simulink model "Reformable_AI"  (R2026a)
settings: Solver=ode23t  StopTime=10  FixedStep=0.01
InitFcn:
  | load('PV_Params_Stage1.mat'); load('PV_Params_Stage2.mat');
values from neighbouring files (symbols this model uses):
  Eg = 1.12    [PV_Params_Stage1.mat]    (also in reformable_AI.m)
  Gref = 1000    [PV_Params_Stage1.mat]    (also in reformable_AI.m)
  I0_ref = 3.04931718656e-08    [PV_Params_Stage1.mat]    (also in reformable_AI.m = exp(x_sol(3)))
  Iph_ref = 1.82004673012    [PV_Params_Stage1.mat]    (also in reformable_AI.m = x_sol(2))
  k_Iph = 0.2    [PV_Params_Stage2.mat]    (also in reformable_AI.m)
  k_Q = 0.2    [reformable_AI.m]
  k_R0 = 0.5    [reformable_AI.m]
  k_R1 = 0.6    [reformable_AI.m]
  k_Rs = 0.5    [PV_Params_Stage2.mat]    (also in reformable_AI.m)
  k_Rsh = 0.6    [PV_Params_Stage2.mat]    (also in reformable_AI.m)
  Ki = 0.0006    [PV_Params_Stage1.mat]    (also in reformable_AI.m)
  n = 1.3    [PV_Params_Stage1.mat]    (also in reformable_AI.m)
  Ns = 36    [PV_Params_Stage1.mat]    (also in reformable_AI.m)
  OCV_tbl = [11.6 11.8 11.9 12.1 12.2 12.3 12.4 12.5 12.6 12.7 12.8]    [Battery_Param_Definition.m]    (also in Battery_Params_Stage3.mat; reformable_AI.m)
  Q = 7    [Battery_Param_Definition.m]    (also in Battery_Params_Stage3.mat; reformable_AI.m)
  R0 = 0.03    [Battery_Param_Definition.m]    (also in Battery_Params_Stage3.mat; reformable_AI.m)
  R1 = 0.015    [Battery_Param_Definition.m]    (also in Battery_Params_Stage3.mat; reformable_AI.m)
  Rs = 0.0128377802072    [PV_Params_Stage1.mat]    (also in reformable_AI.m = x(1))
  Rsh = 500    [PV_Params_Stage1.mat]    (also in reformable_AI.m)
  SOC_bp = [0 10 20 30 40 50 60 70 80 90 100]    [Battery_Param_Definition.m]    (also in Battery_Params_Stage3.mat; reformable_AI.m)
  SOC_init = 100    [Battery_Param_Definition.m]    (also in Battery_Params_Stage3.mat; reformable_AI.m)
  T_life = 25    [PV_Params_Stage2.mat]    (also in reformable_AI.m)
  T_life_batt = 10    [reformable_AI.m]
  Tref = 298.15    [PV_Params_Stage1.mat]    (also in reformable_AI.m)
libraries: fl_lib x6, nesl_utility x5, ee_lib_for_power_systems x1
settings Model: Creator=inspiredkhalid  LastModifiedBy=inspiredkhalid

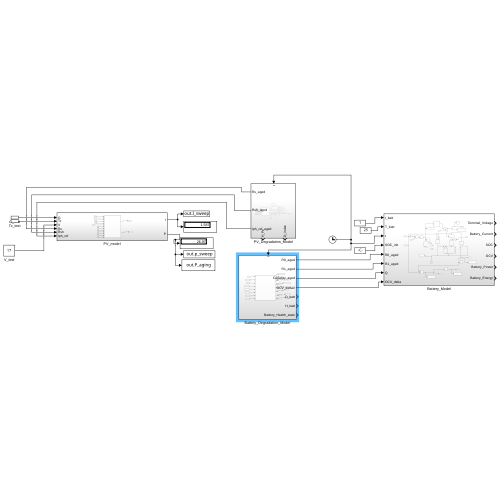
[thumbnail: Simulink's stored preview of the top-level diagram]
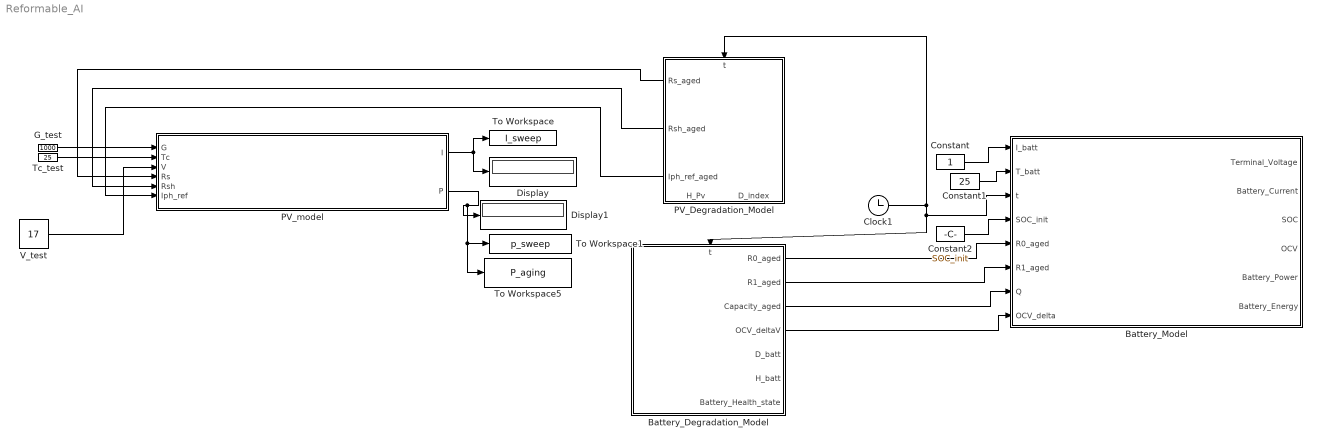
== system Reformable_AI ==
  Battery_Degradation_Model : Subsystem
      settings: PortSchema="{\"entries\":[{\"content\":{\"sides\":[{\"content\":{},\"type\":\"ConnectorPlacement.EquallySpacedRectSide\",\"uuid\":\"1b4fcb6b-66e9-48a9-b94c-f37550c0d7a8\"},{\"content\":{\"connectorIds\":[\"Out1\",\"Out2\",\"Out3\",\"Out4\",\"Out5\",\"Out6\",\"Out7\"],\"side\":\"RIGHT\"},\"type\":\"ConnectorPlacement.EquallySpacedRectSide\",\"uuid\":\"dcdb6d26-adba-4e3a-bfcc-7c50a5c7991f\"},{\"content\":{\"connectorIds\":[\"In1\"],\"side\":\"TOP\"},\"type\":\"ConnectorPlacement.EquallySpacedRectSide\",\"uuid\":\"b25d0552-795d-45d8-a626-a317e68fea8d\"}]},\"type\":\"ConnectorPlacement.EquallySpacedConnector\",\"uuid\":\"9e5bfc09-0161-4367-81be-9c2477d62c24\"}],\"packageUris\":[\"http://schema.mathworks.com/mf0/Connector/R2020b\"],\"version\":\"1.0\"}"
  Battery_Model : Subsystem
  Clock1 : Clock
  Constant : Constant
  Constant1 : Constant  Value=25
  Constant2 : Constant  Value=SOC_init
  Display : Display
  Display1 : Display
  G_test : Constant  Value=1000
  PV_Degradation_Model : Subsystem
      settings: PortSchema="{\"entries\":[{\"content\":{\"sides\":[{\"content\":{\"connectorIds\":[\"In1\"]},\"type\":\"ConnectorPlacement.EquallySpacedRectSide\",\"uuid\":\"fc7c08a7-a329-47c9-9fc8-bd6d0c7412cb\"},{\"content\":{\"connectorIds\":[\"Out1\",\"Out2\"],\"side\":\"RIGHT\"},\"type\":\"ConnectorPlacement.EquallySpacedRectSide\",\"uuid\":\"35a8a444-8a75-40e2-9eb4-ed34268f54da\"},{\"content\":{\"side\":\"TOP\"},\"type\":\"ConnectorPlacement.EquallySpacedRectSide\",\"uuid\":\"f1c409b4-d5ab-4e1c-b6d7-466c0f3dffa6\"},{\"content\":{\"connectorIds\":[\"Out3\",\"Out4\",\"Out5\"],\"side\":\"BOTTOM\"},\"type\":\"ConnectorPlacement.EquallySpacedRectSide\",\"uuid\":\"bca27c1f-7244-4b7d-89ff-49c1beb40a94\"}]},\"type\":\"ConnectorPlacement.EquallySpacedConnector\",\"uuid\":\"e415782b-02d5-4f08-91bd-00003c3592e4\"}],\"packageUris\":[\"http://schema.mathworks.com/mf0/Connector/R2020b\"],\"version\":\"1.0\"}"
  PV_model : Subsystem
  Tc_test : Constant  Value=25
  To Workspace : ToWorkspace  VariableName=I_sweep  SaveFormat=Timeseries  SampleTime=-1
  To Workspace1 : ToWorkspace  VariableName=p_sweep  SaveFormat=Timeseries  SampleTime=-1
  To Workspace5 : ToWorkspace  VariableName=P_aging  SaveFormat=Timeseries  SampleTime=-1
  V_test : Constant  Value=17
  wires:
  G_test/1 -> PV_model/1(G)
  Tc_test/1 -> PV_model/2(Tc)
  PV_model/1(I) -> To Workspace/1, Display/1
  PV_model/2(P) -> Display1/1, To Workspace1/1, To Workspace5/1
  Clock1/1 -> Battery_Degradation_Model/1(t), Battery_Model/3(t), PV_Degradation_Model/1(t)
  V_test/1 -> PV_model/3(V)
  PV_Degradation_Model/3(Rs_aged) -> PV_model/4(Rs)
  PV_Degradation_Model/4(Rsh_aged) -> PV_model/5(Rsh)
  PV_Degradation_Model/5(Iph_ref_aged) -> PV_model/6(Iph_ref)
  Constant1/1 -> Battery_Model/2(T_batt)
  Constant2/1 -> Battery_Model/4(SOC_init)
  Constant/1 -> Battery_Model/1(I_batt)
  Battery_Degradation_Model/1(R0_aged) -> Battery_Model/5(R0_aged)
  Battery_Degradation_Model/2(R1_aged) -> Battery_Model/6(R1_aged)
  Battery_Degradation_Model/3(Capacity_aged) -> Battery_Model/7(Q)
  Battery_Degradation_Model/4(OCV_deltaV) -> Battery_Model/8(OCV_delta)

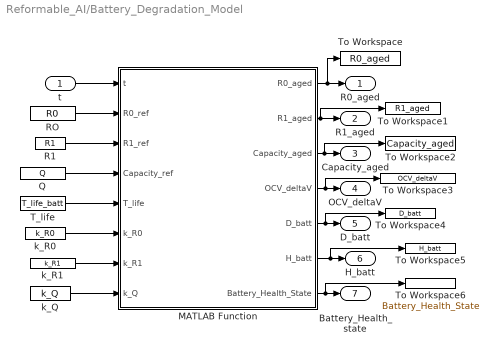
== system Reformable_AI/Battery_Degradation_Model ==
  t : Inport
  MATLAB Function : MATLAB Function  TreatAsAtomicUnit=on
  Q : Constant  Value=Q
  R1 : Constant  Value=R1
  RO : Constant  Value=R0
  T_life : Constant  Value=T_life_batt
  To Workspace : ToWorkspace  VariableName=R0_aged  SaveFormat=Timeseries  SampleTime=-1
  To Workspace1 : ToWorkspace  VariableName=R1_aged  SaveFormat=Timeseries  SampleTime=-1
  To Workspace2 : ToWorkspace  VariableName=Capacity_aged  SaveFormat=Timeseries  SampleTime=-1
  To Workspace3 : ToWorkspace  VariableName=OCV_deltaV  SaveFormat=Timeseries  SampleTime=-1
  To Workspace4 : ToWorkspace  VariableName=D_batt  SaveFormat=Timeseries  SampleTime=-1
  To Workspace5 : ToWorkspace  VariableName=H_batt  SaveFormat=Timeseries  SampleTime=-1
  To Workspace6 : ToWorkspace  VariableName=Battery_Health_State  SaveFormat=Timeseries  SampleTime=-1
  k_Q : Constant  Value=k_Q
  k_R0 : Constant  Value=k_R0
  k_R1 : Constant  Value=k_R1
  R0_aged : Outport
  R1_aged : Outport  Port=2
  Capacity_aged : Outport  Port=3
  OCV_deltaV : Outport  Port=4
  D_batt : Outport  Port=5
  H_batt : Outport  Port=6
  Battery_Health_state : Outport  Port=7
  wires:
  t/1 -> MATLAB Function/1(t)
  RO/1 -> MATLAB Function/2(R0_ref)
  R1/1 -> MATLAB Function/3(R1_ref)
  Q/1 -> MATLAB Function/4(Capacity_ref)
  T_life/1 -> MATLAB Function/5(T_life)
  k_R0/1 -> MATLAB Function/6(k_R0)
  k_R1/1 -> MATLAB Function/7(k_R1)
  k_Q/1 -> MATLAB Function/8(k_Q)
  MATLAB Function/1(R0_aged) -> To Workspace/1, R0_aged/1
  MATLAB Function/2(R1_aged) -> To Workspace1/1, R1_aged/1
  MATLAB Function/3(Capacity_aged) -> To Workspace2/1, Capacity_aged/1
  MATLAB Function/4(OCV_deltaV) -> To Workspace3/1, OCV_deltaV/1
  MATLAB Function/5(D_batt) -> To Workspace4/1, D_batt/1
  MATLAB Function/6(H_batt) -> To Workspace5/1, H_batt/1
  MATLAB Function/7(Battery_Health_State) -> To Workspace6/1, Battery_Health_state/1

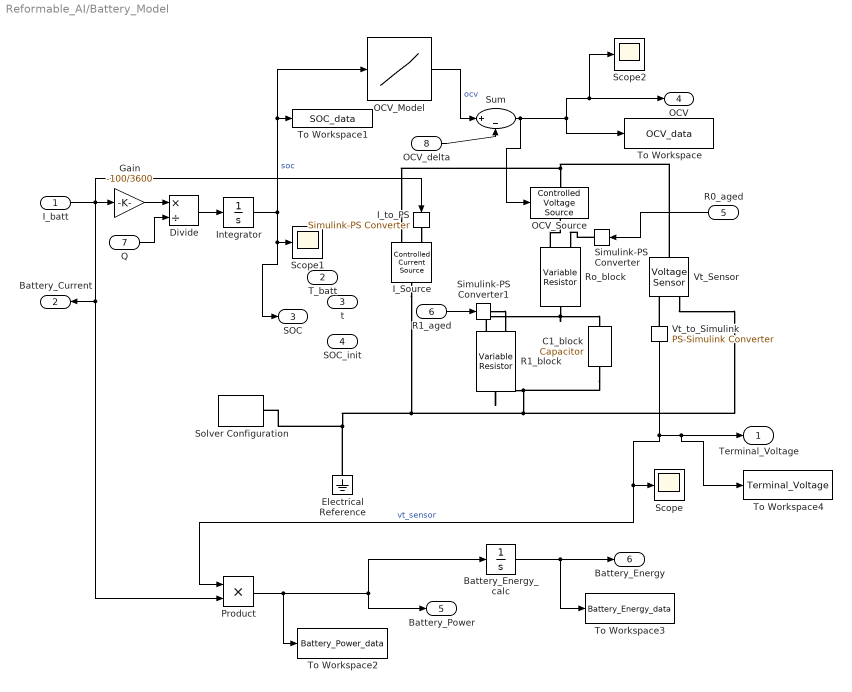
== system Reformable_AI/Battery_Model ==
  I_batt : Inport
  T_batt : Inport  Port=2
  t : Inport  Port=3
  SOC_init : Inport  Port=4
  R0_aged : Inport  Port=5
  R1_aged : Inport  Port=6
  Q : Inport  Port=7
  OCV_delta : Inport  Port=8
  Battery_Energy_calc : Integrator
  C1_block : fl_lib/Electrical/Electrical Elements/Capacitor  c=C1 F  r=1e-6 Ohm  g=0 1/Ohm  i_specify=off  i_priority=None  i=0 A  i_nominal_specify=off  i_nominal_value=1  i_nominal_unit=A  v_specify=off  v_priority=None  v=0 V  v_nominal_specify=off  v_nominal_value=1  v_nominal_unit=V  vc_specify=off  vc_priority=High  vc=0 V  vc_nominal_specify=off  vc_nominal_value=1  vc_nominal_unit=V
  Divide : Product  Inputs=*/
  Electrical Reference : fl_lib/Electrical/Electrical Elements/Electrical Reference
  Gain : Gain  Gain=-100/3600
  I_Source : fl_lib/Electrical/Electrical Sources/Controlled Current Source
  I_to_PS : nesl_utility/Simulink-PS Converter  PhysicalDomain=network_engine_domain  SubClassName=ps_input  LeftPortType=input  RightPortType=output  PseudoPeriodic=off  Frequencies=[]  NoiseDistribution=none  NoiseParameters=[]  Unit=1  AffineConversion=off  FilteringAndDerivatives=provide  SimscapeFilterOrder=1  InputFilterTimeConstant=0.001  UdotUserProvided=0
  Integrator : Integrator  InitialCondition=SOC_init  LimitOutput=on  UpperSaturationLimit=100  LowerSaturationLimit=0
  OCV_Model : Lookup_n-D  NumberOfTableDimensions=1  BreakpointsForDimension1=SOC_bp  Table=OCV_tbl  InternalRulePriority=Speed  RndMeth=Simplest
  OCV_Source : ee_lib_for_power_systems/Sources/Controlled Voltage Source  SystemSampleTime=-1  VariantActivationTime=update diagram  EmptyChoice=off  PassThrough=off  PassThroughVariantControl=(default)  EmptyChoiceVariantControl=(default)  AllowFlexibleInterface=on  Latency=0  AutoFrameSizeCalculation=off
      settings: SourceProductName=Support Library for Power Systems  PortSchema="{\"entries\":[{\"content\":{\"sides\":[{\"content\":{\"connectorIds\":[\"In1\"]},\"type\":\"ConnectorPlacement.EquallySpacedRectSide\",\"uuid\":\"090b2ee3-4378-4784-ad56-1af8514f6806\"},{\"content\":{\"side\":\"RIGHT\"},\"type\":\"ConnectorPlacement.EquallySpacedRectSide\",\"uuid\":\"4adbd240-d61e-4082-b4ef-02f0dbd361b1\"},{\"content\":{\"connectorIds\":[\"LConn1\"],\"side\":\"TOP\"},\"type\":\"ConnectorPlacement.EquallySpacedRectSide\",\"uuid\":\"34d099db-9580-46ff-aa35-d8c98d9402ef\"},{\"content\":{\"connectorIds\":[\"RConn1\"],\"side\":\"BOTTOM\"},\"type\":\"ConnectorPlacement.EquallySpacedRectSide\",\"uuid\":\"ff207868-e9a4-4c5d-8c6f-607ccff15d02\"}]},\"type\":\"ConnectorPlacement.EquallySpacedConnector\",\"uuid\":\"cb3dc6bb-ab47-4bf2-a22f-b68fe84c97d5\"}],\"packageUris\":[\"http://schema.mathworks.com/mf0/Connector/R2020b\"],\"version\":\"1.0\"}"
  Product : Product
  R1_block : fl_lib/Electrical/Electrical Elements/Variable Resistor  Rmin=0 Ohm  thermalEnable=false  thermal_mass=1 J/K  i_specify=off  i_priority=None  i=0 A  i_nominal_specify=off  i_nominal_value=1  i_nominal_unit=A  v_specify=off  v_priority=None  v=0 V  v_nominal_specify=off  v_nominal_value=1  v_nominal_unit=V  T_specify=off  T_priority=None  T=300 K  T_nominal_specify=off  T_nominal_value=1  T_nominal_unit=K
  Ro_block : fl_lib/Electrical/Electrical Elements/Variable Resistor  Rmin=0 Ohm  thermalEnable=false  thermal_mass=1 J/K  i_specify=off  i_priority=None  i=0 A  i_nominal_specify=off  i_nominal_value=1  i_nominal_unit=A  v_specify=off  v_priority=None  v=0 V  v_nominal_specify=off  v_nominal_value=1  v_nominal_unit=V  T_specify=off  T_priority=None  T=300 K  T_nominal_specify=off  T_nominal_value=1  T_nominal_unit=K
  Scope : Scope
      settings: ActiveDisplayYMinimum=-1  ActiveDisplayYMaximum=1
  Scope1 : Scope
      settings: ActiveDisplayYMinimum=99.3303571428569  ActiveDisplayYMaximum=100.07440476190479
  Scope2 : Scope
      settings: ActiveDisplayYMinimum=2.8000000000000007  ActiveDisplayYMaximum=22.8  DataLoggingVariableName=ScopeData2
  Simulink-PS Converter : nesl_utility/Simulink-PS Converter  PhysicalDomain=network_engine_domain  SubClassName=ps_input  LeftPortType=input  RightPortType=output  PseudoPeriodic=off  Frequencies=[]  NoiseDistribution=none  NoiseParameters=[]  Unit=1  AffineConversion=off  FilteringAndDerivatives=provide  SimscapeFilterOrder=1  InputFilterTimeConstant=0.001  UdotUserProvided=0
  Simulink-PS Converter1 : nesl_utility/Simulink-PS Converter  PhysicalDomain=network_engine_domain  SubClassName=ps_input  LeftPortType=input  RightPortType=output  PseudoPeriodic=off  Frequencies=[]  NoiseDistribution=none  NoiseParameters=[]  Unit=1  AffineConversion=off  FilteringAndDerivatives=provide  SimscapeFilterOrder=1  InputFilterTimeConstant=0.001  UdotUserProvided=0
  Solver Configuration : nesl_utility/Solver Configuration  PhysicalDomain=network_engine_domain  SubClassName=solver  LeftPortType=input  RightPortType=generic  Tones=[]  Harmonics=[]  SimulateNoise=off  Profile=off  UseLocalSampling=off  EnableSwitchedLinearOptims=on  FrequencyDomain=off  UseCCode=off  RelTol=0.001  AbsTol=0.001  MinStep=1e-09  ToWorkspace=off  RevertToSquareIcSolve=off  NumHomotopyIterations=100  PhasorMode=off  PhasorModeNumHarmonics=1  ConsistencySolver=NEWTON_XTOL_AFTER_FTOL  CanonicalOrdering=CANONICAL  OptimizeIntermediates=OPTIMIZED  IndexReductionMethod=DerivativeReplacement  DoDC=off  ResidualTolerance=1e-09  ConsistencyTolSource=GLOBAL  ConsistencyAbsTol=0.001  ConsistencyRelTol=0.001  ConsistencyTolFactor=0.001  UseLocalSolver=off  LocalSolverChoice=NE_BACKWARD_EULER_ADVANCER  ResolveIndetEquations=on  FunctionEvalNumThread=1  LocalSolverSampleTime=0.001  DoFixedCost=off  MaxNonlinIter=3  MaxModeIter=2  ComputeImpulses=off  ImpulseIterations=2  LinearAlgebra=auto  LinearAlgebraNumThread=0  EquationFormulation=NE_TIME_EF  DelaysMemoryBudget=1024  AutomaticFiltering=on  FilteringTimeConstant=0.001  PartitionStorageMethod=AS_NEEDED  PartitionMemoryBudget=1024  PartitionMethod=ROBUST  MultibodyUseLocalSolver=off  MultibodyLocalSolverChoice=ODE1  MultibodyLocalSolverSampleTime=0.001
  Sum : Sum  Inputs=|+-
  To Workspace : ToWorkspace  VariableName=OCV_data  SaveFormat=Timeseries  SampleTime=-1
  To Workspace1 : ToWorkspace  VariableName=SOC_data  SaveFormat=Timeseries  SampleTime=-1
  To Workspace2 : ToWorkspace  VariableName=Battery_Power_data  SaveFormat=Timeseries  SampleTime=-1
  To Workspace3 : ToWorkspace  VariableName=Battery_Energy_data  SaveFormat=Timeseries  SampleTime=-1
  To Workspace4 : ToWorkspace  VariableName=Terminal_Voltage  SaveFormat=Timeseries  SampleTime=-1
  Vt_Sensor : fl_lib/Electrical/Electrical Sensors/Voltage Sensor
  Vt_to_Simulink : nesl_utility/PS-Simulink Converter  PhysicalDomain=network_engine_domain  SubClassName=ps_output  LeftPortType=input  RightPortType=output  PseudoPeriodic=off  Frequencies=[]  VectorFormat=inherit  Unit=inherit  AffineConversion=off
  Terminal_Voltage : Outport
  Battery_Current : Outport  Port=2
  SOC : Outport  Port=3
  OCV : Outport  Port=4
  Battery_Power : Outport  Port=5
  Battery_Energy : Outport  Port=6
  wires:
  Vt_to_Simulink/1 -> Product/1, Scope/1, To Workspace4/1, Terminal_Voltage/1  "vt_sensor"
  I_batt/1 -> Gain/1, I_to_PS/1, Product/2, Battery_Current/1
  Integrator/1 -> To Workspace1/1, OCV_Model/1, Scope1/1, SOC/1  "soc"
  OCV_Model/1 -> Sum/1  "ocv"
  Product/1 -> To Workspace2/1, Battery_Energy_calc/1, Battery_Power/1
  Battery_Energy_calc/1 -> To Workspace3/1, Battery_Energy/1
  R0_aged/1 -> Simulink-PS Converter/1
  R1_aged/1 -> Simulink-PS Converter1/1
  Divide/1 -> Integrator/1
  Gain/1 -> Divide/1
  Q/1 -> Divide/2
  Sum/1 -> OCV_Source/1, Scope2/1, OCV/1, To Workspace/1
  OCV_delta/1 -> Sum/2
  connections:
  C1_block/RConn1 -- R1_block/RConn1 -- Vt_Sensor/RConn2 -- Electrical Reference/LConn1 -- Solver Configuration/RConn1 -- I_Source/LConn1
  Ro_block/LConn2 -- OCV_Source/RConn1
  Ro_block/RConn1 -- C1_block/LConn1 -- R1_block/LConn2
  Vt_Sensor/LConn1 -- I_Source/RConn2 -- OCV_Source/LConn1
  Vt_to_Simulink/LConn1 -- Vt_Sensor/RConn1
  I_to_PS/RConn1 -- I_Source/RConn1
  Simulink-PS Converter/RConn1 -- Ro_block/LConn1
  Simulink-PS Converter1/RConn1 -- R1_block/LConn1

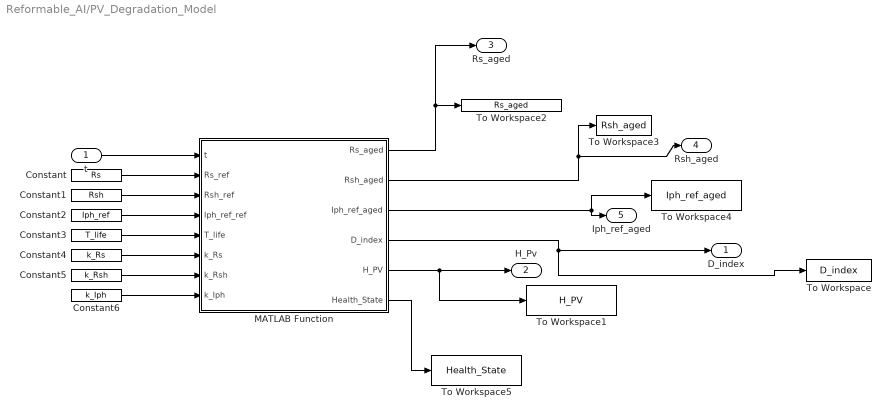
== system Reformable_AI/PV_Degradation_Model ==
  t : Inport
  Constant : Constant  Value=Rs
  Constant1 : Constant  Value=Rsh
  Constant2 : Constant  Value=Iph_ref
  Constant3 : Constant  Value=T_life
  Constant4 : Constant  Value=k_Rs
  Constant5 : Constant  Value=k_Rsh
  Constant6 : Constant  Value=k_Iph
  MATLAB Function : MATLAB Function  TreatAsAtomicUnit=on
  To Workspace : ToWorkspace  VariableName=D_index  SaveFormat=Timeseries  SampleTime=-1
  To Workspace1 : ToWorkspace  VariableName=H_PV  SaveFormat=Timeseries  SampleTime=-1
  To Workspace2 : ToWorkspace  VariableName=Rs_aged  SaveFormat=Timeseries  SampleTime=-1
  To Workspace3 : ToWorkspace  VariableName=Rsh_aged  SaveFormat=Timeseries  SampleTime=-1
  To Workspace4 : ToWorkspace  VariableName=Iph_ref_aged  SaveFormat=Timeseries  SampleTime=-1
  To Workspace5 : ToWorkspace  VariableName=Health_State  SaveFormat=Timeseries  SampleTime=-1
  D_index : Outport
  H_Pv : Outport  Port=2
  Rs_aged : Outport  Port=3
  Rsh_aged : Outport  Port=4
  Iph_ref_aged : Outport  Port=5
  wires:
  t/1 -> MATLAB Function/1(t)
  Constant/1 -> MATLAB Function/2(Rs_ref)
  Constant1/1 -> MATLAB Function/3(Rsh_ref)
  Constant2/1 -> MATLAB Function/4(Iph_ref_ref)
  Constant3/1 -> MATLAB Function/5(T_life)
  Constant4/1 -> MATLAB Function/6(k_Rs)
  Constant5/1 -> MATLAB Function/7(k_Rsh)
  Constant6/1 -> MATLAB Function/8(k_Iph)
  MATLAB Function/2(Rsh_aged) -> To Workspace3/1, Rsh_aged/1
  MATLAB Function/3(Iph_ref_aged) -> Iph_ref_aged/1, To Workspace4/1
  MATLAB Function/4(D_index) -> To Workspace/1, D_index/1
  MATLAB Function/5(H_PV) -> To Workspace1/1, H_Pv/1
  MATLAB Function/1(Rs_aged) -> Rs_aged/1, To Workspace2/1
  MATLAB Function/6(Health_State) -> To Workspace5/1

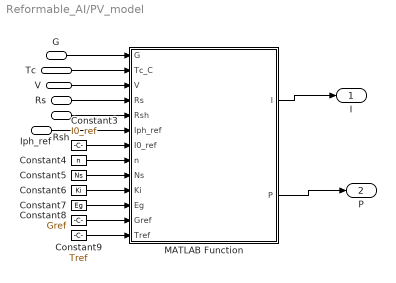
== system Reformable_AI/PV_model ==
  G : Inport
  Tc : Inport  Port=2
  V : Inport  Port=3
  Rs : Inport  Port=4
  Rsh : Inport  Port=5
  Iph_ref : Inport  Port=6
  Constant3 : Constant  Value=I0_ref
  Constant4 : Constant  Value=n
  Constant5 : Constant  Value=Ns
  Constant6 : Constant  Value=Ki
  Constant7 : Constant  Value=Eg
  Constant8 : Constant  Value=Gref
  Constant9 : Constant  Value=Tref
  MATLAB Function : MATLAB Function  TreatAsAtomicUnit=on
  I : Outport
  P : Outport  Port=2
  wires:
  MATLAB Function/1(I) -> I/1
  G/1 -> MATLAB Function/1(G)
  Tc/1 -> MATLAB Function/2(Tc_C)
  V/1 -> MATLAB Function/3(V)
  MATLAB Function/2(P) -> P/1
  Rs/1 -> MATLAB Function/4(Rs)
  Rsh/1 -> MATLAB Function/5(Rsh)
  Iph_ref/1 -> MATLAB Function/6(Iph_ref)
  Constant3/1 -> MATLAB Function/7(I0_ref)
  Constant4/1 -> MATLAB Function/8(n)
  Constant5/1 -> MATLAB Function/9(Ns)
  Constant6/1 -> MATLAB Function/10(Ki)
  Constant7/1 -> MATLAB Function/11(Eg)
  Constant9/1 -> MATLAB Function/13(Tref)
  Constant8/1 -> MATLAB Function/12(Gref)

== matlab function Reformable_AI/PV_Degradation_Model/MATLAB Function ==
  data: t input; Rs_aged output; Rs_ref input; Rsh_ref input; Iph_ref_ref input; T_life input; k_Rs input; k_Rsh input; k_Iph input; Rsh_aged output; Iph_ref_aged output; D_index output; H_PV output; Health_State output

function [Rs_aged, Rsh_aged, Iph_ref_aged, D_index, H_PV, Health_State] = PV_Aging_Model(t, Rs_ref, Rsh_ref, Iph_ref_ref, T_life, k_Rs, k_Rsh, k_Iph)
%#codegen

D_index = min(1, t / T_life);

Rs_aged      = Rs_ref * (1 + k_Rs * D_index);
Rsh_aged     = Rsh_ref * (1 - k_Rsh * D_index);
Iph_ref_aged = Iph_ref_ref * (1 - k_Iph * D_index);

H_PV = 1 - D_index;

% Discrete health state classification (1=Healthy ... 5=Critical)
if D_index < 0.2
    Health_State = 1;   % Healthy
elseif D_index < 0.4
    Health_State = 2;   % Early Degradation
elseif D_index < 0.6
    Health_State = 3;   % Moderate Degradation
elseif D_index < 0.8
    Health_State = 4;   % Severe Degradation
else
    Health_State = 5;   % Critical
end

end

== matlab function Reformable_AI/PV_model/MATLAB Function ==
  data: G input; I output; Tc_C input; V input; Rs input; P output; Rsh input; Iph_ref input; I0_ref input; n input; Ns input; Ki input; Eg input; Gref input; Tref input
function [I, P] = PV_SingleDiode_Solver(G, Tc_C, V, Rs, Rsh, Iph_ref, I0_ref, n, Ns, Ki, Eg, Gref, Tref)
%#codegen

k = 1.380649e-23;
q = 1.602176634e-19;

Tc = Tc_C + 273.15;
Vt = Ns*k*Tc/q;

Iph = (Iph_ref + Ki*(Tc - Tref)) * (G/Gref);
I0  = I0_ref * (Tc/Tref)^3 * exp((q*Eg/(n*k)) * (1/Tref - 1/Tc));

I = Iph;
for iter = 1:50
    expTerm = exp(min((V + I*Rs)/(n*Vt), 700));
    f  = Iph - I0*(expTerm - 1) - (V + I*Rs)/Rsh - I;
    df = -I0*(Rs/(n*Vt))*expTerm - Rs/Rsh - 1;
    dI = f/df;
    I  = I - dI;
    if abs(dI) < 1e-8
        break;
    end
end

I = max(I, 0);
P = V * I;
end

== matlab function Reformable_AI/Battery_Degradation_Model/MATLAB Function ==
  data: t input; R0_aged output; R0_ref input; R1_ref input; Capacity_ref input; T_life input; k_R0 input; k_R1 input; k_Q input; R1_aged output; Capacity_aged output; OCV_deltaV output; D_batt output; H_batt output; Battery_Health_State output
function [R0_aged, R1_aged, Capacity_aged, OCV_deltaV, D_batt, H_batt, Battery_Health_State] = ...
    Battery_Aging_Model(t, R0_ref, R1_ref, Capacity_ref, T_life, k_R0, k_R1, k_Q)
%#codegen

D_batt = min(1, t / T_life);

R0_aged       = R0_ref * (1 + k_R0 * D_batt);
R1_aged       = R1_ref * (1 + k_R1 * D_batt);
Capacity_aged = Capacity_ref * (1 - k_Q * D_batt);

% Small, gradual OCV shift — capped so it never causes a sudden collapse
OCV_deltaV = 0.05 * D_batt;   % up to 50 mV shift at end-of-life; tune if needed

H_batt = 1 - D_batt;

% Discrete health state classification (1=Healthy ... 5=Critical)
if D_batt < 0.2
    Battery_Health_State = 1;
elseif D_batt < 0.4
    Battery_Health_State = 2;
elseif D_batt < 0.6
    Battery_Health_State = 3;
elseif D_batt < 0.8
    Battery_Health_State = 4;
else
    Battery_Health_State = 5;
end

end
